simulink model "hw6"  (R2024a)
settings: Solver=VariableStepAuto  StartTime=0.0  StopTime=10.0  RelTol=1e-3
values from neighbouring files (symbols this model uses):
  u_bar = 1.89    [hw6main.m]
  y = 8    [hw6main.m]
settings Model: Creator=xinchen  LastModifiedBy=xinchen

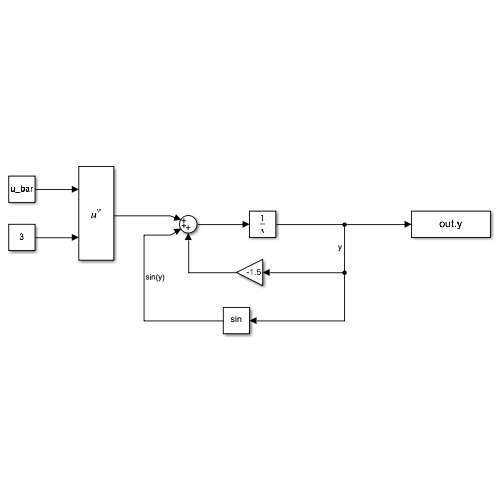
[thumbnail: Simulink's stored preview of the top-level diagram]
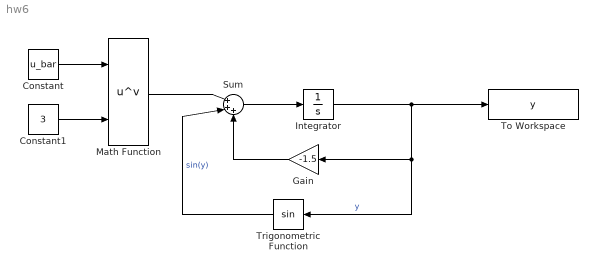
== system hw6 ==
  Constant : Constant  Value=u_bar
  Constant1 : Constant  Value=3
  Gain : Gain  Gain=-1.5
  Integrator : Integrator  InitialCondition=y
  Math Function : Math  Operator=pow
  Sum : Sum  Inputs=|+++
  To Workspace : ToWorkspace  VariableName=y  SampleTime=-1
  Trigonometric Function : Trigonometry
  wires:
  Constant/1 -> Math Function/1
  Math Function/1 -> Sum/1
  Constant1/1 -> Math Function/2
  Trigonometric Function/1 -> Sum/2  "sin(y)"
  Integrator/1 -> To Workspace/1, Trigonometric Function/1, Gain/1  "y"
  Sum/1 -> Integrator/1
  Gain/1 -> Sum/3
